simulink model "gm_soc_dvbs2_fpga"  (R2025b)
settings: Solver=VariableStepAuto  StartTime=0.0  StopTime=10.0  RelTol=1e-3
InitFcn:
  | soc_dvbs2_init;
undefined symbols (not defined in the file or in its folder): Add, coefficientsLog, coefficientsSqrt1, coefficientsSqrt2, dataBits, Deinterleaver, designMultirateFIR, noisePow, Shift, Short, soc_dvbs2_designFIRFilter, soc_dvbs2_txPacketBits, syncWord, txDataOut, txFiltCoeff, XData
libraries: simulink x304, hdlsllib x265, dspsigops x15, dsphdlfiltering2 x8, hdlmdlgenlib x6, dsphdlsigops2 x5, commseqgen3 x5, dsphdlmathfun2 x3, hwlogicconnlib x2, whdledac x2, commhdlcrc x2, whdlutilities x1
(part 14 of 36)

== system gm_soc_dvbs2_fpga/DVBS2/DVBS2 TxRx/DVB-S2 HDL Receiver/Synchronizer and PL Header Decoder/Time Frequency and Coarse Phase Synchronizer/Pilot Blks Counter ==
  pilotIdx : Inport  OutDataTypeStr=fixdt(0, 11, 0)  PortDimensions=1  SampleTime=2.5e-07
  pilotValid : Inport  Port=2  OutDataTypeStr=boolean  PortDimensions=1  SampleTime=2.5e-07
  Compare To Constant : simulink/Logic and Bit Operations/Compare To Constant  relop===  const=config.PilotMinIdx  OutDataTypeStr=boolean
  Delay{1..4} (4 alike) : Delay  DelayLength=1
  HDL Counter : hdlsllib/Sources/HDL Counter  CountType=Free running  CountInit=0  CountStep=1  CountMax=25  CountFromType=Initial value  CountFrom=0  CountResetPort=off  CountLoadPort=off  CountEnbPort=on  CountDirPort=off  CountHitOutputPort=off  CountDataType=Unsigned  CountWordLen=16  CountFracLen=0  CountSampTime=1
  Logical Operator : Logic  AllPortsSameDT=off  OutDataTypeStr=boolean
  pilotBlkCount : Outport  SampleTime=2.5e-07
  wires:
  Delay1/1 -> Compare To Constant/1
  pilotIdx/1 -> Delay1/1
  Delay2/1 -> Logical Operator/2
  pilotValid/1 -> Delay2/1
  Compare To Constant/1 -> Logical Operator/1
  Logical Operator/1 -> Delay4/1
  Delay4/1 -> HDL Counter/1
  HDL Counter/1 -> Delay3/1
  Delay3/1 -> pilotBlkCount/1

== system gm_soc_dvbs2_fpga/DVBS2/DVBS2 TxRx/DVB-S2 HDL Receiver/Synchronizer and PL Header Decoder/Time Frequency and Coarse Phase Synchronizer/Time and Coarse Frequency Synchronizer ==
  dataIn : Inport  OutDataTypeStr=fixdt(1, 18, 15)  PortDimensions=1  SampleTime=6.25e-08
      settings: SignalType=complex
  validIn : Inport  Port=2  OutDataTypeStr=boolean  PortDimensions=1  SampleTime=6.25e-08
  Coarse Frequency Estimator : Subsystem
  Delay{1..4,14} (5 alike) : Delay  DelayLength=double(2)  InitialCondition=0  SampleTime=6.25e-08
  Delay10 : Delay  DelayLength=double(21)  InitialCondition=0  SampleTime=2.5e-07
  Delay11 : Delay  DelayLength=double(26)  InitialCondition=0  SampleTime=2.5e-07
  Delay{28..32,34} (6 alike) : Delay  DelayLength=double(1)  InitialCondition=0  SampleTime=2.5e-07
  Delay5 : Delay  DelayLength=double(1)  InitialCondition=0  SampleTime=6.25e-08
  Delay6 : Delay  DelayLength=double(1)  InitialCondition=0  SampleTime=6.25e-08
  Delay7 : Delay  DelayLength=double(2)  InitialCondition=0  SampleTime=2.5e-07
  Delay8 : Delay  DelayLength=double(2)  InitialCondition=0  SampleTime=2.5e-07
  Delay9 : Delay  DelayLength=double(2)  InitialCondition=0  SampleTime=2.5e-07
  Frame Synchronizer : Subsystem
  Math Function : Math  Operator=conj  OutDataTypeStr=fixdt(1, 16, 14)
  PL Data Descrambler and Pilot Valid Indicator : Subsystem
  Product : Product  Inputs=**  OutDataTypeStr=fixdt(1, 18, 15)  SampleTime=6.25e-08
  RRC Receive Matched Filter : dsphdlfiltering2/Discrete FIR Filter  NumeratorSource=Property  Numerator=config.RRCImpulseResponse  NumeratorPrototype=[]  FilterStructure=Direct form systolic  SerializationOption=Minimum number of cycles between valid input samples  NumCycles=2  NumberOfMultipliers=2  SimulateUsing=Code generation  roundingMode=Floor  overflowMode=off  CoefficientsDataTypeStr=Inherit: Same word length as input  OutputDataTypeStr=Inherit: Same word length as input  ResetInputPort=off  HDLGlobalReset=off  CoeffMultiplier=Multiplier  UseMultForPow2Coeff=on  FrameInputSymmOptim=off
  Symbol Synchronizer : Subsystem
  rstCCFO : Constant  OutDataTypeStr=boolean  SampleTime=2.5e-07
  VisualizeCorrelationSignals : Outport
  normCoarFreqEst : Outport  Port=2  SampleTime=2.5e-07
  symbSyncDataOut : Outport  Port=3  SampleTime=2.5e-07
  symbSyncValidOut : Outport  Port=4  SampleTime=2.5e-07
  pilotIdx : Outport  Port=5  SampleTime=2.5e-07
  pilotValid : Outport  Port=6  SampleTime=2.5e-07
  dataOut : Outport  Port=7  SampleTime=2.5e-07
  validOut : Outport  Port=8  SampleTime=2.5e-07
  endOfSOF : Outport  Port=9  SampleTime=2.5e-07
  hasPilots : Outport  Port=10  SampleTime=2.5e-07
  wires:
  Frame Synchronizer/3(endOfSOF) -> PL Data Descrambler and Pilot Valid Indicator/3(endOfSOFIn)
  dataIn/1 -> Delay3/1
  rstCCFO/1 -> Coarse Frequency Estimator/1(rst)
  PL Data Descrambler and Pilot Valid Indicator/3(dataOut) -> Delay30/1
  Delay14/1 -> RRC Receive Matched Filter/1
  Delay3/1 -> Product/1
  Delay5/1 -> Delay2/1
  PL Data Descrambler and Pilot Valid Indicator/2(pilotValid) -> Delay29/1
  Delay2/1 -> Product/2
  Delay1/1 -> Delay4/1
  Product/1 -> Delay14/1
  validIn/1 -> Delay1/1
  Delay4/1 -> RRC Receive Matched Filter/2
  Math Function/1 -> Delay5/1
  RRC Receive Matched Filter/1 -> Symbol Synchronizer/1(dataIn)
  Delay31/1 -> validOut/1
  RRC Receive Matched Filter/2 -> Symbol Synchronizer/2(validIn)
  Symbol Synchronizer/1(dataOut) -> symbSyncDataOut/1, Frame Synchronizer/1(dataIn)
  Symbol Synchronizer/2(validOut) -> symbSyncValidOut/1, Frame Synchronizer/2(validIn)
  Frame Synchronizer/1(dataOut) -> PL Data Descrambler and Pilot Valid Indicator/1(dataIn)
  Frame Synchronizer/2(validOut) -> PL Data Descrambler and Pilot Valid Indicator/2(validIn)
  Delay7/1 -> Coarse Frequency Estimator/2(dataIn)
  Frame Synchronizer/4(hasPilots) -> Delay10/1, PL Data Descrambler and Pilot Valid Indicator/4(hasPilots)
  Frame Synchronizer/5(VisualizeCorrelationSignals) -> VisualizeCorrelationSignals/1
  PL Data Descrambler and Pilot Valid Indicator/1(pilotidx) -> Delay28/1
  Delay34/1 -> hasPilots/1
  PL Data Descrambler and Pilot Valid Indicator/4(validOut) -> Delay31/1
  PL Data Descrambler and Pilot Valid Indicator/5(endOfSOF) -> Delay32/1
  Delay10/1 -> Delay11/1
  Delay28/1 -> pilotIdx/1, Delay9/1
  Delay29/1 -> Delay8/1, pilotValid/1
  Delay30/1 -> dataOut/1, Delay7/1
  Delay32/1 -> endOfSOF/1
  Delay11/1 -> Delay34/1
  Delay9/1 -> Coarse Frequency Estimator/4(pilotIdx)
  Delay8/1 -> Coarse Frequency Estimator/3(pilotValid)
  Coarse Frequency Estimator/1(complexEstimate) -> Delay6/1
  Coarse Frequency Estimator/2(normFreqEst) -> normCoarFreqEst/1
  Delay6/1 -> Math Function/1

== system gm_soc_dvbs2_fpga/DVBS2/DVBS2 TxRx/DVB-S2 HDL Receiver/Synchronizer and PL Header Decoder/Time Frequency and Coarse Phase Synchronizer/Variance Estimator ==
  dataIn : Inport  OutDataTypeStr=fixdt(1, 18, 13)  PortDimensions=1  SampleTime=2.5e-07
      settings: SignalType=complex
  validIn : Inport  Port=2  OutDataTypeStr=boolean  PortDimensions=1  SampleTime=2.5e-07
  endOfSOFIn : Inport  Port=3  OutDataTypeStr=boolean  PortDimensions=1  SampleTime=2.5e-07
  Delay{11..16} (6 alike) : Delay
  Delay{2..4,18..20,24..26} (9 alike) : Delay  DelayLength=1
  Delay27 : Delay  DelayLength=4
  Delay28 : Delay  DelayLength=4
  Delay29 : Delay  DelayLength=4
  dataOut : Outport  SampleTime=2.5e-07
  validOut : Outport  Port=2  SampleTime=2.5e-07
  endOfSOF : Outport  Port=3  SampleTime=2.5e-07
  wires:
  Delay20/1 -> Delay15/1
  Delay12/1 -> Delay24/1
  endOfSOFIn/1 -> Delay2/1
  dataIn/1 -> Delay4/1
  validIn/1 -> Delay3/1
  Delay4/1 -> Delay18/1
  Delay13/1 -> Delay25/1
  Delay18/1 -> Delay11/1
  Delay2/1 -> Delay20/1
  Delay3/1 -> Delay19/1
  Delay19/1 -> Delay14/1
  Delay11/1 -> Delay12/1
  Delay15/1 -> Delay16/1
  Delay14/1 -> Delay13/1
  Delay16/1 -> Delay26/1
  Delay24/1 -> Delay27/1
  Delay26/1 -> Delay29/1
  Delay25/1 -> Delay28/1
  Delay27/1 -> dataOut/1
  Delay29/1 -> endOfSOF/1
  Delay28/1 -> validOut/1

== system gm_soc_dvbs2_fpga/DVBS2/DVBS2 TxRx/LUT Based Tx/Subsystem1/Subsystem/txLUT1 ==
  rst : Inport  OutDataTypeStr=boolean  PortDimensions=1  SampleTime=2.5e-07
  enb : Inport  Port=2  OutDataTypeStr=boolean  PortDimensions=1  SampleTime=2.5e-07
  1-D Lookup Table : Subsystem
  Compare To Constant : simulink/Logic and Bit Operations/Compare To Constant  relop===  const="fi(0,0,14,0,\"hex\",\"20b0\")"  OutDataTypeStr=boolean
  HDL Counter : hdlsllib/Sources/HDL Counter  CountType=Count limited  CountInit=0  CountStep=1  CountMax=length(DataLUT)-1  CountFromType=Initial value  CountFrom=0  CountResetPort=on  CountLoadPort=off  CountEnbPort=on  CountDirPort=off  CountHitOutputPort=off  CountDataType=Unsigned  CountWordLen=nextpow2(length(DataLUT)-1)  CountFracLen=0  CountSampTime=1
  Out1 : Outport  SampleTime=2.5e-07
  endOfLUT : Outport  Port=2  SampleTime=2.5e-07
  wires:
  rst/1 -> HDL Counter/1
  enb/1 -> HDL Counter/2
  HDL Counter/1 -> Compare To Constant/1, 1-D Lookup Table/1(In1)
  1-D Lookup Table/1(Out1) -> Out1/1
  Compare To Constant/1 -> endOfLUT/1

== system gm_soc_dvbs2_fpga/DVBS2/DVBS2 TxRx/LUT Based Tx/Subsystem1/Subsystem/txLUT2 ==
  rst : Inport  OutDataTypeStr=boolean  PortDimensions=1  SampleTime=2.5e-07
  enb : Inport  Port=2  OutDataTypeStr=boolean  PortDimensions=1  SampleTime=2.5e-07
  1-D Lookup Table : Subsystem
  Compare To Constant : simulink/Logic and Bit Operations/Compare To Constant  relop===  const="fi(0,0,14,0,\"hex\",\"20b0\")"  OutDataTypeStr=boolean
  HDL Counter : hdlsllib/Sources/HDL Counter  CountType=Count limited  CountInit=0  CountStep=1  CountMax=length(DataLUT)-1  CountFromType=Initial value  CountFrom=0  CountResetPort=on  CountLoadPort=off  CountEnbPort=on  CountDirPort=off  CountHitOutputPort=off  CountDataType=Unsigned  CountWordLen=nextpow2(length(DataLUT)-1)  CountFracLen=0  CountSampTime=1
  Out1 : Outport  SampleTime=2.5e-07
  endOfLUT : Outport  Port=2  SampleTime=2.5e-07
  wires:
  rst/1 -> HDL Counter/1
  HDL Counter/1 -> Compare To Constant/1, 1-D Lookup Table/1(In1)
  enb/1 -> HDL Counter/2
  1-D Lookup Table/1(Out1) -> Out1/1
  Compare To Constant/1 -> endOfLUT/1

== system gm_soc_dvbs2_fpga/DVBS2/DVBS2 TxRx/LUT Based Tx/Subsystem1/Subsystem/txLUT3 ==
  rst : Inport  OutDataTypeStr=boolean  PortDimensions=1  SampleTime=2.5e-07
  enb : Inport  Port=2  OutDataTypeStr=boolean  PortDimensions=1  SampleTime=2.5e-07
  1-D Lookup Table : Subsystem
  Compare To Constant : simulink/Logic and Bit Operations/Compare To Constant  relop===  const="fi(0,0,14,0,\"hex\",\"20b0\")"  OutDataTypeStr=boolean
  HDL Counter : hdlsllib/Sources/HDL Counter  CountType=Count limited  CountInit=0  CountStep=1  CountMax=length(DataLUT)-1  CountFromType=Initial value  CountFrom=0  CountResetPort=on  CountLoadPort=off  CountEnbPort=on  CountDirPort=off  CountHitOutputPort=off  CountDataType=Unsigned  CountWordLen=nextpow2(length(DataLUT)-1)  CountFracLen=0  CountSampTime=1
  Out1 : Outport  SampleTime=2.5e-07
  endOfLUT : Outport  Port=2  SampleTime=2.5e-07
  wires:
  rst/1 -> HDL Counter/1
  enb/1 -> HDL Counter/2
  HDL Counter/1 -> Compare To Constant/1, 1-D Lookup Table/1(In1)
  1-D Lookup Table/1(Out1) -> Out1/1
  Compare To Constant/1 -> endOfLUT/1

== system gm_soc_dvbs2_fpga/DVBS2/DVBS2 TxRx/LUT Based Tx/Subsystem1/Subsystem/txLUT4 ==
  rst : Inport  OutDataTypeStr=boolean  PortDimensions=1  SampleTime=2.5e-07
  enb : Inport  Port=2  OutDataTypeStr=boolean  PortDimensions=1  SampleTime=2.5e-07
  1-D Lookup Table : Subsystem
  Compare To Constant : simulink/Logic and Bit Operations/Compare To Constant  relop===  const="fi(0,0,14,0,\"hex\",\"20b0\")"  OutDataTypeStr=boolean
  HDL Counter : hdlsllib/Sources/HDL Counter  CountType=Count limited  CountInit=0  CountStep=1  CountMax=length(DataLUT)-1  CountFromType=Initial value  CountFrom=0  CountResetPort=on  CountLoadPort=off  CountEnbPort=on  CountDirPort=off  CountHitOutputPort=off  CountDataType=Unsigned  CountWordLen=nextpow2(length(DataLUT)-1)  CountFracLen=0  CountSampTime=1
  Out1 : Outport  SampleTime=2.5e-07
  endOfLUT : Outport  Port=2  SampleTime=2.5e-07
  wires:
  rst/1 -> HDL Counter/1
  HDL Counter/1 -> 1-D Lookup Table/1(In1), Compare To Constant/1
  enb/1 -> HDL Counter/2
  1-D Lookup Table/1(Out1) -> Out1/1
  Compare To Constant/1 -> endOfLUT/1

== system gm_soc_dvbs2_fpga/DVBS2/DVBS2 TxRx/LUT Based Tx/Subsystem1/Subsystem/txLUT5 ==
  rst : Inport  OutDataTypeStr=boolean  PortDimensions=1  SampleTime=2.5e-07
  enb : Inport  Port=2  OutDataTypeStr=boolean  PortDimensions=1  SampleTime=2.5e-07
  1-D Lookup Table : Subsystem
  Compare To Constant : simulink/Logic and Bit Operations/Compare To Constant  relop===  const="fi(0,0,14,0,\"hex\",\"20b0\")"  OutDataTypeStr=boolean
  HDL Counter : hdlsllib/Sources/HDL Counter  CountType=Count limited  CountInit=0  CountStep=1  CountMax=length(DataLUT)-1  CountFromType=Initial value  CountFrom=0  CountResetPort=on  CountLoadPort=off  CountEnbPort=on  CountDirPort=off  CountHitOutputPort=off  CountDataType=Unsigned  CountWordLen=nextpow2(length(DataLUT)-1)  CountFracLen=0  CountSampTime=1
  Out1 : Outport  SampleTime=2.5e-07
  endOfLUT : Outport  Port=2  SampleTime=2.5e-07
  wires:
  rst/1 -> HDL Counter/1
  Compare To Constant/1 -> endOfLUT/1
  enb/1 -> HDL Counter/2
  HDL Counter/1 -> Compare To Constant/1, 1-D Lookup Table/1(In1)
  1-D Lookup Table/1(Out1) -> Out1/1

== system gm_soc_dvbs2_fpga/DVBS2/DVBS2 TxRx/LUT Based Tx/Subsystem1/Subsystem/txLUT6 ==
  rst : Inport  OutDataTypeStr=boolean  PortDimensions=1  SampleTime=2.5e-07
  enb : Inport  Port=2  OutDataTypeStr=boolean  PortDimensions=1  SampleTime=2.5e-07
  1-D Lookup Table : Subsystem
  Compare To Constant : simulink/Logic and Bit Operations/Compare To Constant  relop===  const="fi(0,0,14,0,\"hex\",\"20b0\")"  OutDataTypeStr=boolean
  HDL Counter : hdlsllib/Sources/HDL Counter  CountType=Count limited  CountInit=0  CountStep=1  CountMax=length(DataLUT)-1  CountFromType=Initial value  CountFrom=0  CountResetPort=on  CountLoadPort=off  CountEnbPort=on  CountDirPort=off  CountHitOutputPort=off  CountDataType=Unsigned  CountWordLen=nextpow2(length(DataLUT)-1)  CountFracLen=0  CountSampTime=1
  Out1 : Outport  SampleTime=2.5e-07
  endOfLUT : Outport  Port=2  SampleTime=2.5e-07
  wires:
  rst/1 -> HDL Counter/1
  HDL Counter/1 -> Compare To Constant/1, 1-D Lookup Table/1(In1)
  enb/1 -> HDL Counter/2
  1-D Lookup Table/1(Out1) -> Out1/1
  Compare To Constant/1 -> endOfLUT/1

== system gm_soc_dvbs2_fpga/DVBS2/DVBS2 TxRx/LUT Based Tx/Subsystem1/Subsystem1/txLUT1 ==
  rst : Inport  OutDataTypeStr=boolean  PortDimensions=1  SampleTime=2.5e-07
  enb : Inport  Port=2  OutDataTypeStr=boolean  PortDimensions=1  SampleTime=2.5e-07
  1-D Lookup Table : Subsystem
  Compare To Constant : simulink/Logic and Bit Operations/Compare To Constant  relop===  const="fi(0,0,14,0,\"hex\",\"20b0\")"  OutDataTypeStr=boolean
  HDL Counter : hdlsllib/Sources/HDL Counter  CountType=Count limited  CountInit=0  CountStep=1  CountMax=length(DataLUT)-1  CountFromType=Initial value  CountFrom=0  CountResetPort=on  CountLoadPort=off  CountEnbPort=on  CountDirPort=off  CountHitOutputPort=off  CountDataType=Unsigned  CountWordLen=nextpow2(length(DataLUT)-1)  CountFracLen=0  CountSampTime=1
  Out1 : Outport  SampleTime=2.5e-07
  endOfLUT : Outport  Port=2  SampleTime=2.5e-07
  wires:
  rst/1 -> HDL Counter/1
  enb/1 -> HDL Counter/2
  HDL Counter/1 -> Compare To Constant/1, 1-D Lookup Table/1(In1)
  1-D Lookup Table/1(Out1) -> Out1/1
  Compare To Constant/1 -> endOfLUT/1

== system gm_soc_dvbs2_fpga/DVBS2/DVBS2 TxRx/LUT Based Tx/Subsystem1/Subsystem1/txLUT2 ==
  rst : Inport  OutDataTypeStr=boolean  PortDimensions=1  SampleTime=2.5e-07
  enb : Inport  Port=2  OutDataTypeStr=boolean  PortDimensions=1  SampleTime=2.5e-07
  1-D Lookup Table : Subsystem
  Compare To Constant : simulink/Logic and Bit Operations/Compare To Constant  relop===  const="fi(0,0,14,0,\"hex\",\"20b0\")"  OutDataTypeStr=boolean
  HDL Counter : hdlsllib/Sources/HDL Counter  CountType=Count limited  CountInit=0  CountStep=1  CountMax=length(DataLUT)-1  CountFromType=Initial value  CountFrom=0  CountResetPort=on  CountLoadPort=off  CountEnbPort=on  CountDirPort=off  CountHitOutputPort=off  CountDataType=Unsigned  CountWordLen=nextpow2(length(DataLUT)-1)  CountFracLen=0  CountSampTime=1
  Out1 : Outport  SampleTime=2.5e-07
  endOfLUT : Outport  Port=2  SampleTime=2.5e-07
  wires:
  1-D Lookup Table/1(Out1) -> Out1/1
  rst/1 -> HDL Counter/1
  enb/1 -> HDL Counter/2
  HDL Counter/1 -> Compare To Constant/1, 1-D Lookup Table/1(In1)
  Compare To Constant/1 -> endOfLUT/1

== system gm_soc_dvbs2_fpga/DVBS2/DVBS2 TxRx/LUT Based Tx/Subsystem1/Subsystem1/txLUT3 ==
  rst : Inport  OutDataTypeStr=boolean  PortDimensions=1  SampleTime=2.5e-07
  enb : Inport  Port=2  OutDataTypeStr=boolean  PortDimensions=1  SampleTime=2.5e-07
  1-D Lookup Table : Subsystem
  Compare To Constant : simulink/Logic and Bit Operations/Compare To Constant  relop===  const="fi(0,0,14,0,\"hex\",\"20b0\")"  OutDataTypeStr=boolean
  HDL Counter : hdlsllib/Sources/HDL Counter  CountType=Count limited  CountInit=0  CountStep=1  CountMax=length(DataLUT)-1  CountFromType=Initial value  CountFrom=0  CountResetPort=on  CountLoadPort=off  CountEnbPort=on  CountDirPort=off  CountHitOutputPort=off  CountDataType=Unsigned  CountWordLen=nextpow2(length(DataLUT)-1)  CountFracLen=0  CountSampTime=1
  Out1 : Outport  SampleTime=2.5e-07
  endOfLUT : Outport  Port=2  SampleTime=2.5e-07
  wires:
  1-D Lookup Table/1(Out1) -> Out1/1
  rst/1 -> HDL Counter/1
  HDL Counter/1 -> Compare To Constant/1, 1-D Lookup Table/1(In1)
  enb/1 -> HDL Counter/2
  Compare To Constant/1 -> endOfLUT/1

== system gm_soc_dvbs2_fpga/DVBS2/DVBS2 TxRx/LUT Based Tx/Subsystem1/Subsystem1/txLUT4 ==
  rst : Inport  OutDataTypeStr=boolean  PortDimensions=1  SampleTime=2.5e-07
  enb : Inport  Port=2  OutDataTypeStr=boolean  PortDimensions=1  SampleTime=2.5e-07
  1-D Lookup Table : Subsystem
  Compare To Constant : simulink/Logic and Bit Operations/Compare To Constant  relop===  const="fi(0,0,14,0,\"hex\",\"20b1\")"  OutDataTypeStr=boolean
  HDL Counter : hdlsllib/Sources/HDL Counter  CountType=Count limited  CountInit=0  CountStep=1  CountMax=length(DataLUT)-1  CountFromType=Initial value  CountFrom=0  CountResetPort=on  CountLoadPort=off  CountEnbPort=on  CountDirPort=off  CountHitOutputPort=off  CountDataType=Unsigned  CountWordLen=nextpow2(length(DataLUT)-1)  CountFracLen=0  CountSampTime=1
  Out1 : Outport  SampleTime=2.5e-07
  endOfLUT : Outport  Port=2  SampleTime=2.5e-07
  wires:
  rst/1 -> HDL Counter/1
  enb/1 -> HDL Counter/2
  HDL Counter/1 -> Compare To Constant/1, 1-D Lookup Table/1(In1)
  1-D Lookup Table/1(Out1) -> Out1/1
  Compare To Constant/1 -> endOfLUT/1

== system gm_soc_dvbs2_fpga/DVBS2/DVBS2 TxRx/LUT Based Tx/Subsystem1/Subsystem1/txLUT5 ==
  rst : Inport  OutDataTypeStr=boolean  PortDimensions=1  SampleTime=2.5e-07
  enb : Inport  Port=2  OutDataTypeStr=boolean  PortDimensions=1  SampleTime=2.5e-07
  1-D Lookup Table : Subsystem
  Compare To Constant : simulink/Logic and Bit Operations/Compare To Constant  relop===  const="fi(0,0,13,0,\"hex\",\"15dc\")"  OutDataTypeStr=boolean
  HDL Counter : hdlsllib/Sources/HDL Counter  CountType=Count limited  CountInit=0  CountStep=1  CountMax=length(DataLUT)-1  CountFromType=Initial value  CountFrom=0  CountResetPort=on  CountLoadPort=off  CountEnbPort=on  CountDirPort=off  CountHitOutputPort=off  CountDataType=Unsigned  CountWordLen=nextpow2(length(DataLUT)-1)  CountFracLen=0  CountSampTime=1
  Out1 : Outport  SampleTime=2.5e-07
  endOfLUT : Outport  Port=2  SampleTime=2.5e-07
  wires:
  rst/1 -> HDL Counter/1
  enb/1 -> HDL Counter/2
  HDL Counter/1 -> Compare To Constant/1, 1-D Lookup Table/1(In1)
  1-D Lookup Table/1(Out1) -> Out1/1
  Compare To Constant/1 -> endOfLUT/1

== system gm_soc_dvbs2_fpga/DVBS2/DVBS2 TxRx/LUT Based Tx/Subsystem1/Subsystem1/txLUT6 ==
  rst : Inport  OutDataTypeStr=boolean  PortDimensions=1  SampleTime=2.5e-07
  enb : Inport  Port=2  OutDataTypeStr=boolean  PortDimensions=1  SampleTime=2.5e-07
  1-D Lookup Table : Subsystem
  Compare To Constant : simulink/Logic and Bit Operations/Compare To Constant  relop===  const="fi(0,0,13,0,\"hex\",\"15dc\")"  OutDataTypeStr=boolean
  HDL Counter : hdlsllib/Sources/HDL Counter  CountType=Count limited  CountInit=0  CountStep=1  CountMax=length(DataLUT)-1  CountFromType=Initial value  CountFrom=0  CountResetPort=on  CountLoadPort=off  CountEnbPort=on  CountDirPort=off  CountHitOutputPort=off  CountDataType=Unsigned  CountWordLen=nextpow2(length(DataLUT)-1)  CountFracLen=0  CountSampTime=1
  Out1 : Outport  SampleTime=2.5e-07
  endOfLUT : Outport  Port=2  SampleTime=2.5e-07
  wires:
  1-D Lookup Table/1(Out1) -> Out1/1
  rst/1 -> HDL Counter/1
  enb/1 -> HDL Counter/2
  HDL Counter/1 -> Compare To Constant/1, 1-D Lookup Table/1(In1)
  Compare To Constant/1 -> endOfLUT/1

== system gm_soc_dvbs2_fpga/DVBS2/DVBS2 TxRx/LUT Based Tx/Subsystem1/Subsystem2/txLUT1 ==
  rst : Inport  OutDataTypeStr=boolean  PortDimensions=1  SampleTime=2.5e-07
  enb : Inport  Port=2  OutDataTypeStr=boolean  PortDimensions=1  SampleTime=2.5e-07
  1-D Lookup Table : Subsystem
  Compare To Constant : simulink/Logic and Bit Operations/Compare To Constant  relop===  const="fi(0,0,13,0,\"hex\",\"1072\")"  OutDataTypeStr=boolean
  HDL Counter : hdlsllib/Sources/HDL Counter  CountType=Count limited  CountInit=0  CountStep=1  CountMax=length(DataLUT)-1  CountFromType=Initial value  CountFrom=0  CountResetPort=on  CountLoadPort=off  CountEnbPort=on  CountDirPort=off  CountHitOutputPort=off  CountDataType=Unsigned  CountWordLen=nextpow2(length(DataLUT)-1)  CountFracLen=0  CountSampTime=1
  Out1 : Outport  SampleTime=2.5e-07
  endOfLUT : Outport  Port=2  SampleTime=2.5e-07
  wires:
  rst/1 -> HDL Counter/1
  enb/1 -> HDL Counter/2
  HDL Counter/1 -> Compare To Constant/1, 1-D Lookup Table/1(In1)
  1-D Lookup Table/1(Out1) -> Out1/1
  Compare To Constant/1 -> endOfLUT/1

== system gm_soc_dvbs2_fpga/DVBS2/DVBS2 TxRx/LUT Based Tx/Subsystem1/Subsystem2/txLUT2 ==
  rst : Inport  OutDataTypeStr=boolean  PortDimensions=1  SampleTime=2.5e-07
  enb : Inport  Port=2  OutDataTypeStr=boolean  PortDimensions=1  SampleTime=2.5e-07
  1-D Lookup Table : Subsystem
  Compare To Constant : simulink/Logic and Bit Operations/Compare To Constant  relop===  const="fi(0,0,13,0,\"hex\",\"1072\")"  OutDataTypeStr=boolean
  HDL Counter : hdlsllib/Sources/HDL Counter  CountType=Count limited  CountInit=0  CountStep=1  CountMax=length(DataLUT)-1  CountFromType=Initial value  CountFrom=0  CountResetPort=on  CountLoadPort=off  CountEnbPort=on  CountDirPort=off  CountHitOutputPort=off  CountDataType=Unsigned  CountWordLen=nextpow2(length(DataLUT)-1)  CountFracLen=0  CountSampTime=1
  Out1 : Outport  SampleTime=2.5e-07
  endOfLUT : Outport  Port=2  SampleTime=2.5e-07
  wires:
  1-D Lookup Table/1(Out1) -> Out1/1
  rst/1 -> HDL Counter/1
  enb/1 -> HDL Counter/2
  HDL Counter/1 -> 1-D Lookup Table/1(In1), Compare To Constant/1
  Compare To Constant/1 -> endOfLUT/1

== system gm_soc_dvbs2_fpga/DVBS2/DVBS2 TxRx/LUT Based Tx/Subsystem1/Subsystem2/txLUT3 ==
  rst : Inport  OutDataTypeStr=boolean  PortDimensions=1  SampleTime=2.5e-07
  enb : Inport  Port=2  OutDataTypeStr=boolean  PortDimensions=1  SampleTime=2.5e-07
  1-D Lookup Table : Subsystem
  Compare To Constant : simulink/Logic and Bit Operations/Compare To Constant  relop===  const="fi(0,0,12,0,\"hex\",\"d48\")"  OutDataTypeStr=boolean
  HDL Counter : hdlsllib/Sources/HDL Counter  CountType=Count limited  CountInit=0  CountStep=1  CountMax=length(DataLUT)-1  CountFromType=Initial value  CountFrom=0  CountResetPort=on  CountLoadPort=off  CountEnbPort=on  CountDirPort=off  CountHitOutputPort=off  CountDataType=Unsigned  CountWordLen=nextpow2(length(DataLUT)-1)  CountFracLen=0  CountSampTime=1
  Out1 : Outport  SampleTime=2.5e-07
  endOfLUT : Outport  Port=2  SampleTime=2.5e-07
  wires:
  1-D Lookup Table/1(Out1) -> Out1/1
  rst/1 -> HDL Counter/1
  enb/1 -> HDL Counter/2
  Compare To Constant/1 -> endOfLUT/1
  HDL Counter/1 -> Compare To Constant/1, 1-D Lookup Table/1(In1)

== system gm_soc_dvbs2_fpga/DVBS2/DVBS2 TxRx/LUT Based Tx/Subsystem1/Subsystem2/txLUT4 ==
  rst : Inport  OutDataTypeStr=boolean  PortDimensions=1  SampleTime=2.5e-07
  enb : Inport  Port=2  OutDataTypeStr=boolean  PortDimensions=1  SampleTime=2.5e-07
  1-D Lookup Table : Subsystem
  Compare To Constant : simulink/Logic and Bit Operations/Compare To Constant  relop===  const="fi(0,0,12,0,\"hex\",\"d48\")"  OutDataTypeStr=boolean
  HDL Counter : hdlsllib/Sources/HDL Counter  CountType=Count limited  CountInit=0  CountStep=1  CountMax=length(DataLUT)-1  CountFromType=Initial value  CountFrom=0  CountResetPort=on  CountLoadPort=off  CountEnbPort=on  CountDirPort=off  CountHitOutputPort=off  CountDataType=Unsigned  CountWordLen=nextpow2(length(DataLUT)-1)  CountFracLen=0  CountSampTime=1
  Out1 : Outport  SampleTime=2.5e-07
  endOfLUT : Outport  Port=2  SampleTime=2.5e-07
  wires:
  1-D Lookup Table/1(Out1) -> Out1/1
  rst/1 -> HDL Counter/1
  HDL Counter/1 -> 1-D Lookup Table/1(In1), Compare To Constant/1
  enb/1 -> HDL Counter/2
  Compare To Constant/1 -> endOfLUT/1

== system gm_soc_dvbs2_fpga/DVBS2/DVBS2 TxRx/LUT Based Tx/Subsystem1/Subsystem2/txLUT5 ==
  rst : Inport  OutDataTypeStr=boolean  PortDimensions=1  SampleTime=2.5e-07
  enb : Inport  Port=2  OutDataTypeStr=boolean  PortDimensions=1  SampleTime=2.5e-07
  1-D Lookup Table : Subsystem
  Compare To Constant : simulink/Logic and Bit Operations/Compare To Constant  relop===  const="fi(0,0,12,0,\"hex\",\"d48\")"  OutDataTypeStr=boolean
  HDL Counter : hdlsllib/Sources/HDL Counter  CountType=Count limited  CountInit=0  CountStep=1  CountMax=length(DataLUT)-1  CountFromType=Initial value  CountFrom=0  CountResetPort=on  CountLoadPort=off  CountEnbPort=on  CountDirPort=off  CountHitOutputPort=off  CountDataType=Unsigned  CountWordLen=nextpow2(length(DataLUT)-1)  CountFracLen=0  CountSampTime=1
  Out1 : Outport  SampleTime=2.5e-07
  endOfLUT : Outport  Port=2  SampleTime=2.5e-07
  wires:
  rst/1 -> HDL Counter/1
  enb/1 -> HDL Counter/2
  HDL Counter/1 -> 1-D Lookup Table/1(In1), Compare To Constant/1
  1-D Lookup Table/1(Out1) -> Out1/1
  Compare To Constant/1 -> endOfLUT/1

== system gm_soc_dvbs2_fpga/DVBS2/DVBS2 TxRx/LUT Based Tx/Subsystem1/Subsystem2/txLUT6 ==
  rst : Inport  OutDataTypeStr=boolean  PortDimensions=1  SampleTime=2.5e-07
  enb : Inport  Port=2  OutDataTypeStr=boolean  PortDimensions=1  SampleTime=2.5e-07
  1-D Lookup Table : Subsystem
  Compare To Constant : simulink/Logic and Bit Operations/Compare To Constant  relop===  const="fi(0,0,12,0,\"hex\",\"d48\")"  OutDataTypeStr=boolean
  HDL Counter : hdlsllib/Sources/HDL Counter  CountType=Count limited  CountInit=0  CountStep=1  CountMax=length(DataLUT)-1  CountFromType=Initial value  CountFrom=0  CountResetPort=on  CountLoadPort=off  CountEnbPort=on  CountDirPort=off  CountHitOutputPort=off  CountDataType=Unsigned  CountWordLen=nextpow2(length(DataLUT)-1)  CountFracLen=0  CountSampTime=1
  Out1 : Outport  SampleTime=2.5e-07
  endOfLUT : Outport  Port=2  SampleTime=2.5e-07
  wires:
  1-D Lookup Table/1(Out1) -> Out1/1
  rst/1 -> HDL Counter/1
  enb/1 -> HDL Counter/2
  HDL Counter/1 -> Compare To Constant/1, 1-D Lookup Table/1(In1)
  Compare To Constant/1 -> endOfLUT/1

== system gm_soc_dvbs2_fpga/DVBS2/DVBS2 TxRx/LUT Based Tx/Subsystem1/Subsystem4/txLUT1 ==
  rst : Inport  OutDataTypeStr=boolean  PortDimensions=1  SampleTime=2.5e-07
  enb : Inport  Port=2  OutDataTypeStr=boolean  PortDimensions=1  SampleTime=2.5e-07
  1-D Lookup Table : Subsystem
  Compare To Constant : simulink/Logic and Bit Operations/Compare To Constant  relop===  const="fi(0,0,13,0,\"hex\",\"15dc\")"  OutDataTypeStr=boolean
  HDL Counter : hdlsllib/Sources/HDL Counter  CountType=Count limited  CountInit=0  CountStep=1  CountMax=length(DataLUT)-1  CountFromType=Initial value  CountFrom=0  CountResetPort=on  CountLoadPort=off  CountEnbPort=on  CountDirPort=off  CountHitOutputPort=off  CountDataType=Unsigned  CountWordLen=nextpow2(length(DataLUT)-1)  CountFracLen=0  CountSampTime=1
  Out1 : Outport  SampleTime=2.5e-07
  endOfLUT : Outport  Port=2  SampleTime=2.5e-07
  wires:
  rst/1 -> HDL Counter/1
  enb/1 -> HDL Counter/2
  HDL Counter/1 -> Compare To Constant/1, 1-D Lookup Table/1(In1)
  1-D Lookup Table/1(Out1) -> Out1/1
  Compare To Constant/1 -> endOfLUT/1

== system gm_soc_dvbs2_fpga/DVBS2/DVBS2 TxRx/LUT Based Tx/Subsystem1/Subsystem4/txLUT2 ==
  rst : Inport  OutDataTypeStr=boolean  PortDimensions=1  SampleTime=2.5e-07
  enb : Inport  Port=2  OutDataTypeStr=boolean  PortDimensions=1  SampleTime=2.5e-07
  1-D Lookup Table : Subsystem
  Compare To Constant : simulink/Logic and Bit Operations/Compare To Constant  relop===  const="fi(0,0,13,0,\"hex\",\"15dc\")"  OutDataTypeStr=boolean
  HDL Counter : hdlsllib/Sources/HDL Counter  CountType=Count limited  CountInit=0  CountStep=1  CountMax=length(DataLUT)-1  CountFromType=Initial value  CountFrom=0  CountResetPort=on  CountLoadPort=off  CountEnbPort=on  CountDirPort=off  CountHitOutputPort=off  CountDataType=Unsigned  CountWordLen=nextpow2(length(DataLUT)-1)  CountFracLen=0  CountSampTime=1
  Out1 : Outport  SampleTime=2.5e-07
  endOfLUT : Outport  Port=2  SampleTime=2.5e-07
  wires:
  1-D Lookup Table/1(Out1) -> Out1/1
  rst/1 -> HDL Counter/1
  HDL Counter/1 -> 1-D Lookup Table/1(In1), Compare To Constant/1
  enb/1 -> HDL Counter/2
  Compare To Constant/1 -> endOfLUT/1

== system gm_soc_dvbs2_fpga/DVBS2/DVBS2 TxRx/LUT Based Tx/Subsystem1/Subsystem4/txLUT3 ==
  rst : Inport  OutDataTypeStr=boolean  PortDimensions=1  SampleTime=2.5e-07
  enb : Inport  Port=2  OutDataTypeStr=boolean  PortDimensions=1  SampleTime=2.5e-07
  1-D Lookup Table : Subsystem
  Compare To Constant : simulink/Logic and Bit Operations/Compare To Constant  relop===  const="fi(0,0,13,0,\"hex\",\"15dc\")"  OutDataTypeStr=boolean
  HDL Counter : hdlsllib/Sources/HDL Counter  CountType=Count limited  CountInit=0  CountStep=1  CountMax=length(DataLUT)-1  CountFromType=Initial value  CountFrom=0  CountResetPort=on  CountLoadPort=off  CountEnbPort=on  CountDirPort=off  CountHitOutputPort=off  CountDataType=Unsigned  CountWordLen=nextpow2(length(DataLUT)-1)  CountFracLen=0  CountSampTime=1
  Out1 : Outport  SampleTime=2.5e-07
  endOfLUT : Outport  Port=2  SampleTime=2.5e-07
  wires:
  1-D Lookup Table/1(Out1) -> Out1/1
  rst/1 -> HDL Counter/1
  HDL Counter/1 -> Compare To Constant/1, 1-D Lookup Table/1(In1)
  enb/1 -> HDL Counter/2
  Compare To Constant/1 -> endOfLUT/1

== system gm_soc_dvbs2_fpga/DVBS2/DVBS2 TxRx/LUT Based Tx/Subsystem1/Subsystem4/txLUT4 ==
  rst : Inport  OutDataTypeStr=boolean  PortDimensions=1  SampleTime=2.5e-07
  enb : Inport  Port=2  OutDataTypeStr=boolean  PortDimensions=1  SampleTime=2.5e-07
  1-D Lookup Table : Subsystem
  Compare To Constant : simulink/Logic and Bit Operations/Compare To Constant  relop===  const="fi(0,0,13,0,\"hex\",\"1072\")"  OutDataTypeStr=boolean
  HDL Counter : hdlsllib/Sources/HDL Counter  CountType=Count limited  CountInit=0  CountStep=1  CountMax=length(DataLUT)-1  CountFromType=Initial value  CountFrom=0  CountResetPort=on  CountLoadPort=off  CountEnbPort=on  CountDirPort=off  CountHitOutputPort=off  CountDataType=Unsigned  CountWordLen=nextpow2(length(DataLUT)-1)  CountFracLen=0  CountSampTime=1
  Out1 : Outport  SampleTime=2.5e-07
  endOfLUT : Outport  Port=2  SampleTime=2.5e-07
  wires:
  rst/1 -> HDL Counter/1
  enb/1 -> HDL Counter/2
  HDL Counter/1 -> Compare To Constant/1, 1-D Lookup Table/1(In1)
  1-D Lookup Table/1(Out1) -> Out1/1
  Compare To Constant/1 -> endOfLUT/1

== system gm_soc_dvbs2_fpga/DVBS2/DVBS2 TxRx/LUT Based Tx/Subsystem1/Subsystem4/txLUT5 ==
  rst : Inport  OutDataTypeStr=boolean  PortDimensions=1  SampleTime=2.5e-07
  enb : Inport  Port=2  OutDataTypeStr=boolean  PortDimensions=1  SampleTime=2.5e-07
  1-D Lookup Table : Subsystem
  Compare To Constant : simulink/Logic and Bit Operations/Compare To Constant  relop===  const="fi(0,0,13,0,\"hex\",\"1072\")"  OutDataTypeStr=boolean
  HDL Counter : hdlsllib/Sources/HDL Counter  CountType=Count limited  CountInit=0  CountStep=1  CountMax=length(DataLUT)-1  CountFromType=Initial value  CountFrom=0  CountResetPort=on  CountLoadPort=off  CountEnbPort=on  CountDirPort=off  CountHitOutputPort=off  CountDataType=Unsigned  CountWordLen=nextpow2(length(DataLUT)-1)  CountFracLen=0  CountSampTime=1
  Out1 : Outport  SampleTime=2.5e-07
  endOfLUT : Outport  Port=2  SampleTime=2.5e-07
  wires:
  1-D Lookup Table/1(Out1) -> Out1/1
  rst/1 -> HDL Counter/1
  enb/1 -> HDL Counter/2
  HDL Counter/1 -> Compare To Constant/1, 1-D Lookup Table/1(In1)
  Compare To Constant/1 -> endOfLUT/1

== system gm_soc_dvbs2_fpga/DVBS2/DVBS2 TxRx/LUT Based Tx/Subsystem1/Subsystem4/txLUT6 ==
  rst : Inport  OutDataTypeStr=boolean  PortDimensions=1  SampleTime=2.5e-07
  enb : Inport  Port=2  OutDataTypeStr=boolean  PortDimensions=1  SampleTime=2.5e-07
  1-D Lookup Table : Subsystem
  Compare To Constant : simulink/Logic and Bit Operations/Compare To Constant  relop===  const="fi(0,0,13,0,\"hex\",\"1072\")"  OutDataTypeStr=boolean
  HDL Counter : hdlsllib/Sources/HDL Counter  CountType=Count limited  CountInit=0  CountStep=1  CountMax=length(DataLUT)-1  CountFromType=Initial value  CountFrom=0  CountResetPort=on  CountLoadPort=off  CountEnbPort=on  CountDirPort=off  CountHitOutputPort=off  CountDataType=Unsigned  CountWordLen=nextpow2(length(DataLUT)-1)  CountFracLen=0  CountSampTime=1
  Out1 : Outport  SampleTime=2.5e-07
  endOfLUT : Outport  Port=2  SampleTime=2.5e-07
  wires:
  1-D Lookup Table/1(Out1) -> Out1/1
  rst/1 -> HDL Counter/1
  HDL Counter/1 -> Compare To Constant/1, 1-D Lookup Table/1(In1)
  enb/1 -> HDL Counter/2
  Compare To Constant/1 -> endOfLUT/1

== system gm_soc_dvbs2_fpga/DVBS2/DVBS2 TxRx/Channel/AWGN Generator/Unit Variance Gaussian Noise/SinCos/Sine HDL Optimized1 ==
  note: (C) 2016 Mathworks, Inc
  u : Inport  OutDataTypeStr=fixdt(0, 16, 16)  SampleTime=6.25e-08
  1st or 4th Quad : Logic  Operator=OR  AllPortsSameDT=off  OutDataTypeStr=boolean  SampleTime=6.25e-08
  Amp25 : Sum  Inputs=+-  OutDataTypeStr=fixdt(1, 17, 16)  AccumDataTypeStr=fixdt(1, 17, 16)  SampleTime=6.25e-08
  Amp75 : Sum  Inputs=+-  OutDataTypeStr=fixdt(1, 17, 16)  AccumDataTypeStr=fixdt(1, 17, 16)  SampleTime=6.25e-08
  CastU16En1 : DataTypeConversion  OutDataTypeStr=fixdt(0, 12, 0)  ConvertRealWorld=Stored Integer (SI)  SampleTime=6.25e-08  SaturateOnIntegerOverflow=off  RndMeth=Floor
  CastU16En2 : DataTypeConversion  OutDataTypeStr=fixdt(0, 12, 0)  ConvertRealWorld=Stored Integer (SI)  SampleTime=6.25e-08  RndMeth=Floor
  CastU16En3 : DataTypeConversion  OutDataTypeStr=fixdt(0, 13, 0)  SampleTime=6.25e-08  SaturateOnIntegerOverflow=off  RndMeth=Floor
  Cosine : hdlmdlgenlib/Buffer
  GTEp75 : RelationalOperator  OutDataTypeStr=boolean  SampleTime=6.25e-08  InputSameDT=off
  LTEp25 : RelationalOperator  Operator=<=  OutDataTypeStr=boolean  SampleTime=6.25e-08  InputSameDT=off
  LTEp50 : RelationalOperator  Operator=<=  OutDataTypeStr=boolean  SampleTime=6.25e-08  InputSameDT=off
  Look-Up Table : Subsystem
  Negate : UnaryMinus  SampleTime=6.25e-08
  Point25 : Constant  Value=0.25  OutDataTypeStr=fixdt(0, 16, 16)  SampleTime=6.25e-08
  Point50 : Constant  Value=0.5  OutDataTypeStr=fixdt(0, 16, 16)  SampleTime=6.25e-08
  Point75 : Constant  Value=0.75  OutDataTypeStr=fixdt(0, 16, 16)  SampleTime=6.25e-08
  Positive : DataTypeConversion  OutDataTypeStr=fixdt('sfix16_En15')
  QuadHandle1a : Switch  Criteria=u2 ~= 0  Threshold="fi(0,0,1,0,\"hex\",\"0\")"  OutDataTypeStr=fixdt(1, 17, 16)  SampleTime=6.25e-08  SaturateOnIntegerOverflow=off  InputSameDT=off
  QuadHandle1b : Switch  Criteria=u2 ~= 0  Threshold="fi(0,0,1,0,\"hex\",\"0\")"  OutDataTypeStr=fixdt(1, 17, 16)  SampleTime=6.25e-08  SaturateOnIntegerOverflow=off  InputSameDT=off
  QuadHandle2 : Switch  Criteria=u2 ~= 0  Threshold="fi(0,0,1,0,\"hex\",\"0\")"  OutDataTypeStr=fixdt(0, 12, 12)  SampleTime=6.25e-08  InputSameDT=off
  RAMDelayBalance : hdlmdlgenlib/Buffer
  Saturation : Saturate  UpperLimit="fi(0,0,12,0,\"hex\",\"3ff\")"  LowerLimit="fi(0,0,12,0,\"hex\",\"000\")"  SampleTime=6.25e-08  OutDataTypeStr=fixdt(0, 12, 0)
  SignCorrected : Switch  Criteria=u2 ~= 0  Threshold="fi(0,0,8,0,\"hex\",\"00\")"  OutDataTypeStr=fixdt(1, 16, 15)  SampleTime=6.25e-08  SaturateOnIntegerOverflow=off  InputSameDT=off
  Switch : Switch  Criteria=u2 ~= 0  Threshold="fi(0,0,1,0,\"hex\",\"0\")"  OutDataTypeStr=fixdt(0, 12, 0)  SampleTime=6.25e-08  SaturateOnIntegerOverflow=off  InputSameDT=off
  delayMatch : Delay  DelayLength=double(1)  InitialCondition=0  SampleTime=6.25e-08
  dtc : DataTypeConversion  OutDataTypeStr=uint8  ConvertRealWorld=Stored Integer (SI)  SampleTime=6.25e-08  SaturateOnIntegerOverflow=off  RndMeth=Floor
  insig : DataTypeConversion  OutDataTypeStr=fixdt(0, 12, 12)  SampleTime=6.25e-08  SaturateOnIntegerOverflow=off  RndMeth=Floor
  p25mA : Sum  Inputs=+-  OutDataTypeStr=fixdt(1, 17, 16)  AccumDataTypeStr=fixdt(1, 17, 16)  SampleTime=6.25e-08
  p75mA : Sum  Inputs=+-  OutDataTypeStr=fixdt(1, 17, 16)  AccumDataTypeStr=fixdt(1, 17, 16)  SampleTime=6.25e-08
  pow2switch : Constant  OutDataTypeStr=boolean  SampleTime=6.25e-08
  x : Outport  SampleTime=6.25e-08  VectorParamsAs1DForOutWhenUnconnected=off
  wires:
  Point75/1 -> p75mA/1, GTEp75/2, Amp75/2
  u/1 -> insig/1
  Point50/1 -> LTEp50/2
  Point25/1 -> p25mA/1, LTEp25/2, Amp25/2
  p25mA/1 -> QuadHandle1a/1
  SignCorrected/1 -> Cosine/1
  QuadHandle2/1 -> CastU16En1/1
  insig/1 -> p25mA/2, LTEp50/1, LTEp25/1, GTEp75/1, Amp75/1, Amp25/1, p75mA/2
  LTEp50/1 -> QuadHandle2/2
  GTEp75/1 -> 1st or 4th Quad/2, QuadHandle1b/2
  CastU16En3/1 -> CastU16En2/1
  LTEp25/1 -> QuadHandle1a/2, 1st or 4th Quad/1
  Amp25/1 -> QuadHandle1a/3
  Cosine/1 -> x/1
  dtc/1 -> RAMDelayBalance/1
  Amp75/1 -> QuadHandle1b/1
  p75mA/1 -> QuadHandle1b/3
  1st or 4th Quad/1 -> dtc/1
  Negate/1 -> SignCorrected/3
  QuadHandle1a/1 -> QuadHandle2/1
  Saturation/1 -> Switch/1
  QuadHandle1b/1 -> QuadHandle2/3
  RAMDelayBalance/1 -> delayMatch/1
  Positive/1 -> SignCorrected/1
  CastU16En1/1 -> CastU16En3/1
  delayMatch/1 -> SignCorrected/2
  CastU16En2/1 -> Switch/3, Saturation/1
  Look-Up Table/1(Out1) -> Positive/1, Negate/1
  pow2switch/1 -> Switch/2
  Switch/1 -> Look-Up Table/1(In1)

== system gm_soc_dvbs2_fpga/DVBS2/DVBS2 TxRx/Channel/AWGN Generator/Unit Variance Gaussian Noise/SinCos/Sine HDL Optimized2 ==
  note: (C) 2016 Mathworks, Inc
  u : Inport  OutDataTypeStr=fixdt(0, 16, 16)  SampleTime=6.25e-08
  Amp50 : Sum  Inputs=+-  OutDataTypeStr=fixdt(1, 17, 16)  AccumDataTypeStr=fixdt(1, 17, 16)  SampleTime=6.25e-08
  CastU16En2 : DataTypeConversion  OutDataTypeStr=fixdt(0, 12, 0)  ConvertRealWorld=Stored Integer (SI)  SampleTime=6.25e-08  SaturateOnIntegerOverflow=off  RndMeth=Floor
  CastU16En3 : DataTypeConversion  OutDataTypeStr=fixdt(0, 12, 0)  ConvertRealWorld=Stored Integer (SI)  SampleTime=6.25e-08  RndMeth=Floor
  CastU16En4 : DataTypeConversion  OutDataTypeStr=fixdt(0, 13, 0)  SampleTime=6.25e-08  SaturateOnIntegerOverflow=off  RndMeth=Floor
  LTEp25 : RelationalOperator  Operator=<=  OutDataTypeStr=boolean  SampleTime=6.25e-08  InputSameDT=off
  LTEp50 : RelationalOperator  Operator=<=  OutDataTypeStr=boolean  SampleTime=6.25e-08  InputSameDT=off
  Look-Up Table : Subsystem
  Negate : UnaryMinus  SampleTime=6.25e-08
  Point25 : Constant  Value=0.25  OutDataTypeStr=fixdt(0, 16, 16)  SampleTime=6.25e-08
  Point50 : Constant  Value=0.5  OutDataTypeStr=fixdt(0, 16, 16)  SampleTime=6.25e-08
  Positive : DataTypeConversion  OutDataTypeStr=fixdt('sfix16_En15')
  QuadHandle1 : Switch  Criteria=u2 ~= 0  Threshold="fi(0,0,1,0,\"hex\",\"0\")"  OutDataTypeStr=fixdt(1, 17, 16)  SampleTime=6.25e-08  SaturateOnIntegerOverflow=off  InputSameDT=off
  QuadHandle2 : Switch  Criteria=u2 ~= 0  Threshold="fi(0,0,1,0,\"hex\",\"0\")"  OutDataTypeStr=fixdt(0, 12, 12)  SampleTime=6.25e-08  SaturateOnIntegerOverflow=off  InputSameDT=off
  RAMDelayBalance : hdlmdlgenlib/Buffer
  Saturation : Saturate  UpperLimit="fi(0,0,12,0,\"hex\",\"3ff\")"  LowerLimit="fi(0,0,12,0,\"hex\",\"000\")"  SampleTime=6.25e-08  OutDataTypeStr=fixdt(0, 12, 0)
  SignCorrected : Switch  Criteria=u2 ~= 0  Threshold="fi(0,0,1,0,\"hex\",\"0\")"  OutDataTypeStr=fixdt(1, 16, 15)  SampleTime=6.25e-08  SaturateOnIntegerOverflow=off  InputSameDT=off
  Sine : hdlmdlgenlib/Buffer
  Switch : Switch  Criteria=u2 ~= 0  Threshold="fi(0,0,1,0,\"hex\",\"0\")"  OutDataTypeStr=fixdt(0, 12, 0)  SampleTime=6.25e-08  SaturateOnIntegerOverflow=off  InputSameDT=off
  delayMatch : Delay  DelayLength=double(1)  InitialCondition=0  SampleTime=6.25e-08
  insig : DataTypeConversion  OutDataTypeStr=fixdt(0, 12, 12)  SampleTime=6.25e-08  SaturateOnIntegerOverflow=off  RndMeth=Floor
  p50mA : Sum  Inputs=+-  OutDataTypeStr=fixdt(1, 18, 16)  AccumDataTypeStr=fixdt(1, 18, 16)  SampleTime=6.25e-08
  pow2switch : Constant  OutDataTypeStr=boolean  SampleTime=6.25e-08
  x : Outport  SampleTime=6.25e-08  VectorParamsAs1DForOutWhenUnconnected=off
  wires:
  Point25/1 -> LTEp25/2
  u/1 -> insig/1
  Saturation/1 -> Switch/1
  QuadHandle1/1 -> p50mA/2, QuadHandle2/1, LTEp25/1
  SignCorrected/1 -> Sine/1
  QuadHandle2/1 -> CastU16En2/1
  insig/1 -> QuadHandle1/1, LTEp50/1, Amp50/1
  RAMDelayBalance/1 -> delayMatch/1
  Point50/1 -> LTEp50/2, Amp50/2, p50mA/1
  CastU16En4/1 -> CastU16En3/1
  LTEp50/1 -> QuadHandle1/2, RAMDelayBalance/1
  Amp50/1 -> QuadHandle1/3
  LTEp25/1 -> QuadHandle2/2
  p50mA/1 -> QuadHandle2/3
  delayMatch/1 -> SignCorrected/2
  CastU16En2/1 -> CastU16En4/1
  CastU16En3/1 -> Switch/3, Saturation/1
  pow2switch/1 -> Switch/2
  Switch/1 -> Look-Up Table/1(In1)
  Sine/1 -> x/1
  Look-Up Table/1(Out1) -> Positive/1, Negate/1
  Positive/1 -> SignCorrected/1
  Negate/1 -> SignCorrected/3

== system gm_soc_dvbs2_fpga/DVBS2/DVBS2 TxRx/Channel/AWGN Generator/Unit Variance Gaussian Noise/SqrtImplementation/SqrtEval ==
  u : Inport  OutDataTypeStr=fixdt(0, 31, 24)  PortDimensions=1  SampleTime=6.25e-08
  FunctionEvaluation : Subsystem
  RangeReconstruction : Subsystem
  RangeReduction : Subsystem
  f : Outport  SampleTime=6.25e-08
  wires:
  RangeReconstruction/1(f) -> f/1
  u/1 -> RangeReduction/1(u)
  RangeReduction/1(x_f) -> FunctionEvaluation/1(x_f)
  RangeReduction/3(exp_f) -> FunctionEvaluation/3(exp_fIn)
  RangeReduction/2(pass) -> FunctionEvaluation/2(passIn)
  FunctionEvaluation/3(exp_fOut) -> RangeReconstruction/3(exp_f)
  FunctionEvaluation/2(passOut) -> RangeReconstruction/2(pass)
  FunctionEvaluation/1(y_f) -> RangeReconstruction/1(y_f)

== system gm_soc_dvbs2_fpga/DVBS2/DVBS2 TxRx/Channel/AWGN Generator/Unit Variance Gaussian Noise/TausUniformRandGen/ConcatandExtract ==
  a : Inport  OutDataTypeStr=uint32  PortDimensions=1  SampleTime=6.25e-08
  b : Inport  Port=2  OutDataTypeStr=uint32  PortDimensions=1  SampleTime=6.25e-08
  Bit Concat : hdlsllib/Logic and Bit Operations/Bit Concat  numInputs=2
  Bitwise Operator : simulink/Logic and Bit Operations/Bitwise Operator  logicop=AND  UseBitMask=on  BitMask=bin2dec('00000000000000001111111111111111')  BitMaskRealWorld=Stored Integer
  Data Type Conversion : DataTypeConversion  OutDataTypeStr=uint16  SaturateOnIntegerOverflow=off  RndMeth=Floor
  Data Type Conversion2 : DataTypeConversion  OutDataTypeStr=fixdt(0,16,0)  SaturateOnIntegerOverflow=off  RndMeth=Floor
  Shift Arithmetic : ArithShift  BinPtShiftNumber=-16
  Shift Arithmetic1 : ArithShift  BinPtShiftNumber=-48
  Shift Arithmetic2 : ArithShift  BitShiftNumber=16  BitShiftDirection=Right
  u0(48,48) : Outport  SampleTime=6.25e-08
  u1(16,16) : Outport  Port=2  SampleTime=6.25e-08
  wires:
  a/1 -> Bit Concat/1
  b/1 -> Shift Arithmetic2/1, Bitwise Operator/1
  Shift Arithmetic/1 -> u1(16,16)/1
  Bit Concat/1 -> Shift Arithmetic1/1
  Data Type Conversion2/1 -> Shift Arithmetic/1
  Data Type Conversion/1 -> Bit Concat/2
  Bitwise Operator/1 -> Data Type Conversion2/1
  Shift Arithmetic2/1 -> Data Type Conversion/1
  Shift Arithmetic1/1 -> u0(48,48)/1

== system gm_soc_dvbs2_fpga/DVBS2/DVBS2 TxRx/Channel/AWGN Generator/Unit Variance Gaussian Noise/TausUniformRandGen/TausURNG1 ==
  note: S1
  note: S1
  note: S0
  Bit Shift : hdlsllib/Logic and Bit Operations/Bit Shift  mode=Shift Left Logical  N=double(13)
  Bit Shift1 : hdlsllib/Logic and Bit Operations/Bit Shift  mode=Shift Right Logical  N=double(19)
  Bit Shift2 : hdlsllib/Logic and Bit Operations/Bit Shift  mode=Shift Left Logical  N=double(12)
  Bit Shift3 : hdlsllib/Logic and Bit Operations/Bit Shift  mode=Shift Left Logical  N=double(2)
  Bit Shift4 : hdlsllib/Logic and Bit Operations/Bit Shift  mode=Shift Left Logical  N=double(4)
  Bit Shift5 : hdlsllib/Logic and Bit Operations/Bit Shift  mode=Shift Right Logical  N=double(25)
  Bit Shift6 : hdlsllib/Logic and Bit Operations/Bit Shift  mode=Shift Left Logical  N=double(3)
  Bit Shift7 : hdlsllib/Logic and Bit Operations/Bit Shift  mode=Shift Left Logical  N=double(17)
  Bit Shift8 : hdlsllib/Logic and Bit Operations/Bit Shift  mode=Shift Right Logical  N=double(11)
  Bitwise Operator{,2..3,5..6,8} (6 alike) : simulink/Logic and Bit Operations/Bitwise Operator  logicop=XOR  UseBitMask=off  NumInputPorts=2  BitMask=double(0)  BitMaskRealWorld=Real World Value
  Bitwise Operator1 : simulink/Logic and Bit Operations/Bitwise Operator  logicop=AND  UseBitMask=on  BitMask="fi(0,0,32,0,\"hex\",\"fffffffe\")"  BitMaskRealWorld=Real World Value
  Bitwise Operator4 : simulink/Logic and Bit Operations/Bitwise Operator  logicop=AND  UseBitMask=on  BitMask="fi(0,0,32,0,\"hex\",\"fffffff8\")"  BitMaskRealWorld=Real World Value
  Bitwise Operator7 : simulink/Logic and Bit Operations/Bitwise Operator  logicop=AND  UseBitMask=on  BitMask="fi(0,0,32,0,\"hex\",\"fffffff0\")"  BitMaskRealWorld=Real World Value
  Bitwise Operator9 : simulink/Logic and Bit Operations/Bitwise Operator  logicop=XOR  UseBitMask=off  NumInputPorts=3  BitMask=double(0)  BitMaskRealWorld=Real World Value
  Data Type Conversion : DataTypeConversion  OutDataTypeStr=fixdt('uint32')
  Data Type Conversion1 : DataTypeConversion  OutDataTypeStr=fixdt('uint32')
  Data Type Conversion2 : DataTypeConversion  OutDataTypeStr=fixdt('uint32')
  Delay : Delay  DelayLength=double(1)  InitialCondition=121  SampleTime=6.25e-08
  Delay1 : Delay  DelayLength=double(1)  InitialCondition=719  SampleTime=6.25e-08
  Delay2 : Delay  DelayLength=double(1)  InitialCondition=511  SampleTime=6.25e-08
  a : Outport  SampleTime=6.25e-08
  wires:
  Bitwise Operator6/1 -> Bit Shift8/1
  Data Type Conversion/1 -> Bitwise Operator/2, Bitwise Operator1/1, Bit Shift/1
  Bit Shift2/1 -> Bitwise Operator2/2
  Delay/1 -> Data Type Conversion/1
  Bit Shift3/1 -> Bitwise Operator3/1
  Delay1/1 -> Data Type Conversion1/1
  Data Type Conversion2/1 -> Bitwise Operator6/2, Bitwise Operator7/1, Bit Shift6/1
  Bit Shift7/1 -> Bitwise Operator8/2
  Bitwise Operator1/1 -> Bit Shift2/1
  Delay2/1 -> Data Type Conversion2/1
  Data Type Conversion1/1 -> Bitwise Operator3/2, Bitwise Operator4/1, Bit Shift3/1
  Bit Shift/1 -> Bitwise Operator/1
  Bitwise Operator4/1 -> Bit Shift4/1
  Bitwise Operator9/1 -> a/1
  Bit Shift6/1 -> Bitwise Operator6/1
  Bitwise Operator7/1 -> Bit Shift7/1
  Bitwise Operator/1 -> Bit Shift1/1
  Bitwise Operator3/1 -> Bit Shift5/1
  Bit Shift4/1 -> Bitwise Operator5/2
  Bit Shift1/1 -> Bitwise Operator2/1
  Bit Shift5/1 -> Bitwise Operator5/1
  Bit Shift8/1 -> Bitwise Operator8/1
  Bitwise Operator2/1 -> Delay/1, Bitwise Operator9/1
  Bitwise Operator5/1 -> Delay1/1, Bitwise Operator9/2
  Bitwise Operator8/1 -> Delay2/1, Bitwise Operator9/3
